simulink model "part2"  (R2024a)
settings: Solver=VariableStepAuto  StartTime=0.0  StopTime=200  RelTol=1e-3
undefined symbols (not defined in the file or in its folder): magnitude
settings Model: Creator=katutu  LastModifiedBy=katutu

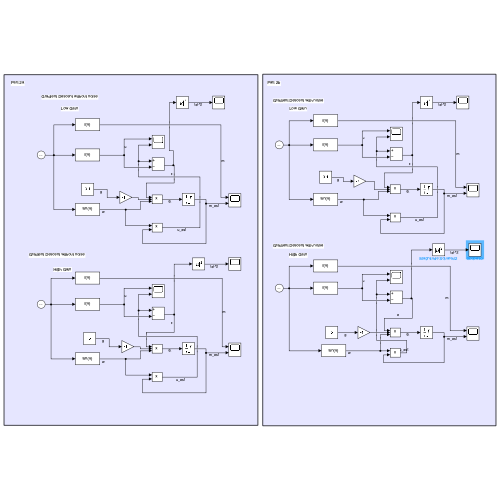
[thumbnail: Simulink's stored preview of the top-level diagram]
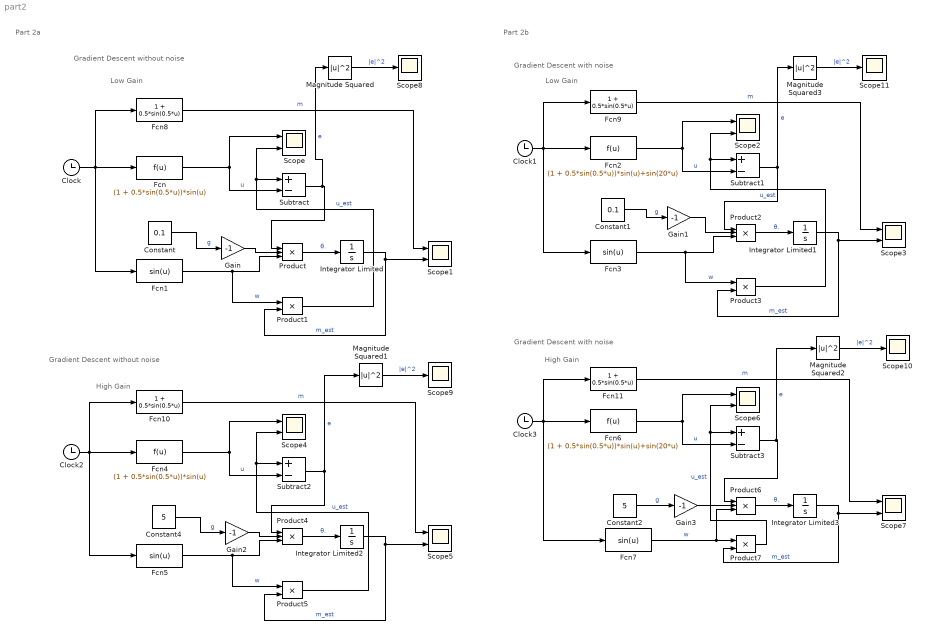
== system part2 ==
  note: Gradient Descent with noise
  note: Part 2a
  note: Low Gain
  note: High Gain
  note: Gradient Descent with noise
  note: High Gain
  note: Part 2b
  note: Gradient Descent without noise
  note: Gradient Descent without noise
  note: Low Gain
  Clock{,1..3} (4 alike) : Clock
  Constant : Constant  Value=0.1
  Constant1 : Constant  Value=0.1
  Constant2 : Constant  Value=5
  Constant4 : Constant  Value=5
  Fcn : Fcn  Expr=(1 + 0.5*sin(0.5*u))*sin(u)
  Fcn{1,3,5,7} (4 alike) : Fcn  Expr=sin(u)
  Fcn{8..11} (4 alike) : Fcn  Expr=1 + 0.5*sin(0.5*u)
  Fcn2 : Fcn  Expr=(1 + 0.5*sin(0.5*u))*sin(u)+sin(20*u)
  Fcn4 : Fcn  Expr=(1 + 0.5*sin(0.5*u))*sin(u)
  Fcn6 : Fcn  Expr=(1 + 0.5*sin(0.5*u))*sin(u)+sin(20*u)
  Gain{,1..3} (4 alike) : Gain  Gain=-1
  Integrator Limited{,1..3} (4 alike) : Integrator  LimitOutput=on  UpperSaturationLimit=10  LowerSaturationLimit=0
  Magnitude Squared{,1..3} (4 alike) : Math  Operator=magnitude^2
  Product{,2,4,6} (4 alike) : Product  Inputs=3
  Product{1,3,5,7} (4 alike) : Product
  Scope{,1..7} (8 alike) : Scope  NumInputPorts=2
  Scope{8..11} (4 alike) : Scope
  Subtract{,1..3} (4 alike) : Sum  Inputs=+-
  wires:
  Subtract3/1 -> Magnitude Squared2/1, Product6/1  "e"
  Product1/1 -> Subtract/1, Scope/2  "u_est"
  Integrator Limited/1 -> Product1/2, Scope1/2  "m_est"
  Product5/1 -> Scope4/2, Subtract2/1  "u_est"
  Clock/1 -> Fcn8/1, Fcn1/1, Fcn/1
  Product/1 -> Integrator Limited/1  "θ."
  Product6/1 -> Integrator Limited3/1  "θ."
  Product3/1 -> Subtract1/1, Scope2/2  "u_est"
  Gain/1 -> Product/2
  Subtract1/1 -> Product2/1, Magnitude Squared3/1  "e"
  Fcn5/1 -> Product5/1, Product4/3  "w"
  Fcn6/1 -> Subtract3/2, Scope6/1  "u"
  Subtract2/1 -> Magnitude Squared1/1, Product4/1  "e"
  Product7/1 -> Subtract3/1, Scope6/2  "u_est"
  Fcn3/1 -> Product3/1, Product2/3  "w"
  Fcn2/1 -> Subtract1/2, Scope2/1  "u"
  Integrator Limited3/1 -> Product7/2, Scope7/2  "m_est"
  Clock2/1 -> Fcn5/1, Fcn10/1, Fcn4/1
  Constant1/1 -> Gain1/1  "g"
  Constant/1 -> Gain/1  "g"
  Fcn7/1 -> Product6/3, Product7/1  "w"
  Product2/1 -> Integrator Limited1/1  "θ."
  Integrator Limited2/1 -> Product5/2, Scope5/2  "m_est"
  Product4/1 -> Integrator Limited2/1  "θ."
  Fcn4/1 -> Subtract2/2, Scope4/1  "u"
  Integrator Limited1/1 -> Product3/2, Scope3/2  "m_est"
  Constant4/1 -> Gain2/1  "g"
  Clock3/1 -> Fcn11/1, Fcn7/1, Fcn6/1
  Constant2/1 -> Gain3/1  "g"
  Clock1/1 -> Fcn9/1, Fcn3/1, Fcn2/1
  Fcn/1 -> Subtract/2, Scope/1  "u"
  Subtract/1 -> Magnitude Squared/1, Product/1  "e"
  Fcn1/1 -> Product1/1, Product/3  "w"
  Gain1/1 -> Product2/2
  Gain3/1 -> Product6/2
  Gain2/1 -> Product4/2
  Fcn8/1 -> Scope1/1  "m"
  Fcn9/1 -> Scope3/1  "m"
  Fcn10/1 -> Scope5/1  "m"
  Fcn11/1 -> Scope7/1  "m"
  Magnitude Squared/1 -> Scope8/1  "|e|^2"
  Magnitude Squared1/1 -> Scope9/1  "|e|^2"
  Magnitude Squared2/1 -> Scope10/1  "|e|^2"
  Magnitude Squared3/1 -> Scope11/1  "|e|^2"
